simulink model "exampleEU_Tapping"  (R2013b)
settings: Solver=ode45  StartTime=0.0  StopTime=24*3600  MaxStep=60  RelTol=1e-3
libraries: carnot x7
settings Model: Creator=drhf  LastModifiedBy=drhf
settings OptimizationCC: ExpressionDepthLimit=2147483647
settings DebuggingCC: StateNameClashWarn=warning
settings GRTTargetCC: CombineOutputUpdateFcns=off  GRTInterface=on

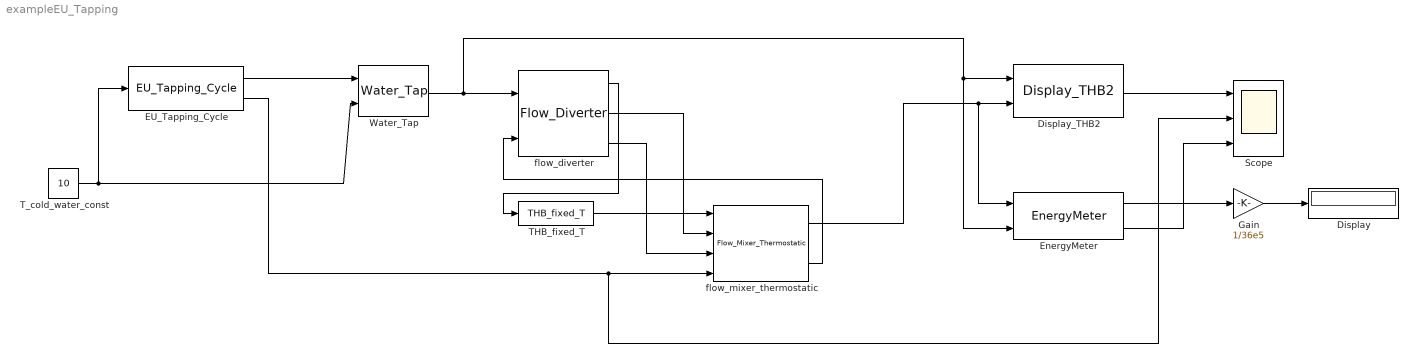
== system exampleEU_Tapping ==
  Display : Display
  Display_THB2 : carnot/Outputs/Display_THB2  t=off  m=on  p=off  id=off  mix=off  d=off
  EU_Tapping_Cycle : carnot/Load/Hot_Water_Tapping/EU_Tapping_Cycle  eu_tap=M
  EnergyMeter : carnot/Control/EnergyMeter
  Gain : Gain  Gain=1/36e5
  Scope : Scope  NumInputPorts=3
      settings: YMin=-5~-5~-5  YMax=5~5~5
  THB_fixed_T : carnot/Source/Simple/THB_fixed_T  t=60
  T_cold_water_const : Constant  Value=10
  Water_Tap : carnot/Load/Hot_Water_Tapping/Water_Tap  dia=0.02  p=2e5
  flow_diverter : carnot/Hydraulics/Flow_Diverter
  flow_mixer_thermostatic : carnot/Hydraulics/Flow_Mixer_Thermostatic  t=10
  wires:
  Display_THB2/1 -> Scope/1
  EnergyMeter/1 -> Gain/1
  Gain/1 -> Display/1
  EnergyMeter/2 -> Scope/3
  Water_Tap/1 -> flow_diverter/1, Display_THB2/1, EnergyMeter/2
  T_cold_water_const/1 -> Water_Tap/2, EU_Tapping_Cycle/1
  EU_Tapping_Cycle/1 -> Water_Tap/1
  EU_Tapping_Cycle/2 -> flow_mixer_thermostatic/4, Scope/2
  flow_diverter/3 -> flow_mixer_thermostatic/3
  flow_diverter/2 -> flow_mixer_thermostatic/2
  THB_fixed_T/1 -> flow_mixer_thermostatic/1
  flow_mixer_thermostatic/1 -> Display_THB2/2, EnergyMeter/1
  flow_mixer_thermostatic/2 -> flow_diverter/2
  flow_diverter/1 -> THB_fixed_T/1
